simulink model "RPI_1"  (R2016a)
settings: Solver=FixedStepDiscrete  StartTime=0.0  StopTime=inf  RelTol=1e-3
libraries: embdlinuxlib x2, visiongeotforms x1
settings Model: SimulationMode=external  ExtModeTrigDuration=100  Creator=The MathWorks, Inc.  LastModifiedBy=Yewly
settings SolverCC: PositivePriorityOrder=on
settings DataIOCC: LimitDataPoints=on  SaveFormat=Array
settings OptimizationCC: ExpressionDepthLimit=2147483647  OptimizeModelRefInitCode=on  LifeSpan=Inf  MaxStackSize=64
settings DebuggingCC: UnderspecifiedInitializationDetection=Classic  MergeDetectMultiDrivingBlocksExec=none  FcnCallInpInsideContextMsg=EnableAllAsWarning  AllowSymbolicDim=off  StateNameClashWarn=warning
settings HardwareCC: ProdBitPerPointer=32  ProdLargestAtomicInteger=Long  ProdLargestAtomicFloat=Double  ProdWordSize=32  ProdHWDeviceType=ARM Compatible->ARM Cortex  UseEmbeddedCoderFeatures=off  UseSimulinkCoderFeatures=off
settings ModelReferenceCC: PropagateSignalLabelsOutOfModel=off
settings RTWCC: SystemTargetFile=ert.tlc  HardwareBoard=Raspberry Pi  TemplateMakefile=ert_default_tmf  GenerateReport=on  RTWVerbose=off  Toolchain=GNU GCC Raspberry Pi  LaunchReport=on
settings CodeAppCC: ForceParamTrailComments=on  IgnoreCustomStorageClasses=off  OperatorAnnotations=on  SimulinkDataObjDesc=on  SFDataObjDesc=on  MATLABFcnDesc=on  CustomSymbolStrType=$N$R$M  InsertBlockDesc=on  MATLABSourceComments=on  InternalIdentifier=Classic
settings ERTTargetCC: SupportNonInlinedSFcns=on
settings ConfigComp: CovModelRefEnable=Off

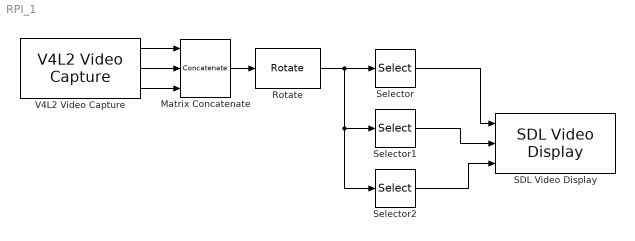
== system RPI_1 ==
  Matrix Concatenate : Concatenate  NumInputs=3  Mode=Multidimensional array  ConcatenateDimension=3
  Rotate : visiongeotforms/Rotate  outSizeR=Expanded to fit rotated input image  src_angle=Specify via dialog  unit_angle=Degrees  angle=pi  maxAngle=pi  dispImage=Center  method=Table lookup  fillVal=0  interpMethod=Bilinear  prodOutputMode=Binary point scaling  prodOutputWordLength=32  prodOutputFracLength=10  roundingMode=Nearest  overflowMode=on
  SDL Video Display : embdlinuxlib/SDL Video Display  pixelFormat=RGB  pixelOrder=Planar  rowMajor=on  blockPlatform=Raspberry Pi
  Selector : Selector  NumberOfDimensions=3  InputPortWidth=3  IndexOptions=Select all,Select all,Index vector (dialog)  Indices=[; ;1],1,1  OutputSizes=1,1,1
  Selector1 : Selector  NumberOfDimensions=3  InputPortWidth=3  IndexOptions=Select all,Select all,Index vector (dialog)  Indices=[; ;1],1,2  OutputSizes=1,1,1
  Selector2 : Selector  NumberOfDimensions=3  InputPortWidth=3  IndexOptions=Select all,Select all,Index vector (dialog)  Indices=[; ;1],1,3  OutputSizes=1,1,1
  V4L2 Video Capture : embdlinuxlib/V4L2 Video Capture  m_devName='/dev/video0'  roi=[0, 0, 640, 480]  imSizeSelection=320x240  imSize=[640, 480]  pixelFormat=RGB  pixelOrder=Planar  sampleTime=1/30  simOutput=Colorbars  blockPlatform=Raspberry Pi
  wires:
  V4L2 Video Capture/1 -> Matrix Concatenate/1
  V4L2 Video Capture/2 -> Matrix Concatenate/2
  V4L2 Video Capture/3 -> Matrix Concatenate/3
  Selector/1 -> SDL Video Display/1
  Matrix Concatenate/1 -> Rotate/1
  Rotate/1 -> Selector2/1, Selector1/1, Selector/1
  Selector2/1 -> SDL Video Display/3
  Selector1/1 -> SDL Video Display/2
